simulink subsystem "Do_Model"  (R2022b)
settings: Solver=VariableStepAuto  StartTime=0.0  StopTime=10.0  RelTol=1e-3
undefined symbols (not defined in the file or in its folder): importedData
libraries: matrix_library x9
settings Model: Creator=hollis  LastModifiedBy=hollis

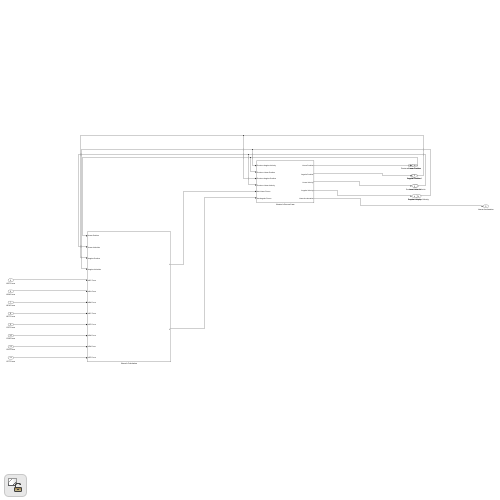
[thumbnail: Simulink's stored preview of the top-level diagram]
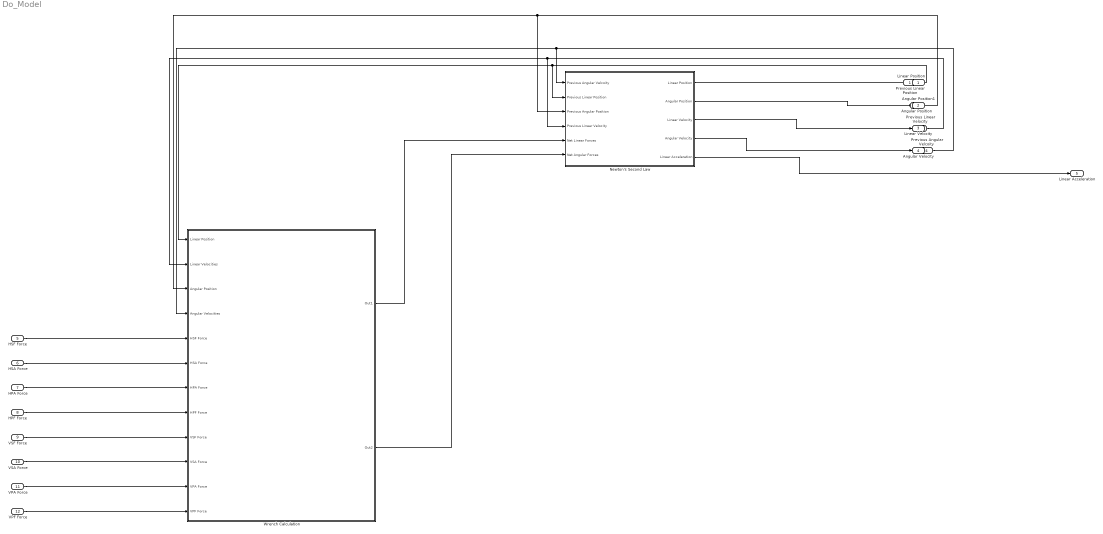
== system Do_Model ==
  Previous Linear Position : Inport
  Angular Position : Inport  Port=2
  Previous Linear Velocity : Inport  Port=3
  Previous Angular Velcoity : Inport  Port=4
  HSF Force : Inport  Port=5
  HSA Force : Inport  Port=6
  HPA Force : Inport  Port=7
  HPF Force : Inport  Port=8
  VSF Force : Inport  Port=9
  VSA Force : Inport  Port=10
  VPA Force : Inport  Port=11
  VPF Force : Inport  Port=12
  Newton's Second Law : Subsystem
  Wrench Calculation : Subsystem
  Linear Position : Outport
  Angular Position1 : Outport  Port=2
  Linear Velocity : Outport  Port=3
  Angular Velocity : Outport  Port=4
  Linear Acceleration : Outport  Port=5
  wires:
  VSF Force/1 -> Wrench Calculation/9(VSF Force)
  Newton's Second Law/3(Linear Velocity) -> Linear Velocity/1
  Wrench Calculation/2(Out2) -> Newton's Second Law/6(Net Angular Forces)
  Newton's Second Law/4(Angular Velocity) -> Angular Velocity/1
  VSA Force/1 -> Wrench Calculation/10(VSA Force)
  Wrench Calculation/1(Out1) -> Newton's Second Law/5(Net Linear Forces)
  HPA Force/1 -> Wrench Calculation/7(HPA Force)
  Previous Angular Velcoity/1 -> Wrench Calculation/4(Angular Velocities), Newton's Second Law/1(Previous Angular Velcoity)
  Newton's Second Law/2(Angular Position) -> Angular Position1/1
  HSA Force/1 -> Wrench Calculation/6(HSA Force)
  VPF Force/1 -> Wrench Calculation/12(VPF Force)
  VPA Force/1 -> Wrench Calculation/11(VPA Force)
  HSF Force/1 -> Wrench Calculation/5(HSF Force)
  Previous Linear Position/1 -> Wrench Calculation/1(Linear Position), Newton's Second Law/2(Previous Linear Position)
  Newton's Second Law/5(Linear Acceleration) -> Linear Acceleration/1
  Angular Position/1 -> Newton's Second Law/3(Previous Angular Position), Wrench Calculation/3(Angular Position)
  Newton's Second Law/1(Linear Position) -> Linear Position/1
  HPF Force/1 -> Wrench Calculation/8(HPF Force)
  Previous Linear Velocity/1 -> Wrench Calculation/2(Linear Velocities), Newton's Second Law/4(Previous Linear Velocity)

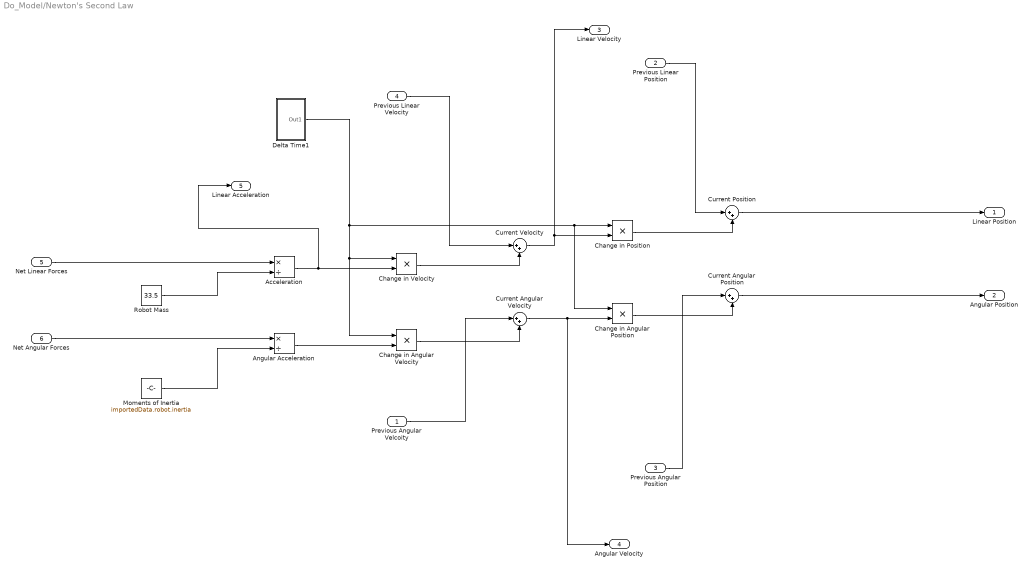
== system Do_Model/Newton's Second Law ==
  Previous Angular Velcoity : Inport
  Previous Linear Position : Inport  Port=2
  Previous Angular Position : Inport  Port=3
  Previous Linear Velocity : Inport  Port=4
  Net Linear Forces : Inport  Port=5
  Net Angular Forces : Inport  Port=6
  Acceleration : Product  Inputs=*/
  Angular Acceleration : Product  Inputs=*/
  Change in Angular Position : Product
  Change in Angular Velocity : Product
  Change in Position : Product
  Change in Velocity : Product
  Current Angular Position : Sum  Inputs=|++
  Current Angular Velocity : Sum  Inputs=|++
  Current Position : Sum  Inputs=|++
  Current Velocity : Sum  Inputs=|++
  Delta Time1 : Subsystem
  Moments of Inertia : Constant  Value=importedData.robot.inertia  VectorParams1D=off
  Robot Mass : Constant  Value=33.5
  Linear Position : Outport
  Angular Position : Outport  Port=2
  Linear Velocity : Outport  Port=3
  Angular Velocity : Outport  Port=4
  Linear Acceleration : Outport  Port=5
  wires:
  Change in Velocity/1 -> Current Velocity/2
  Previous Angular Position/1 -> Current Angular Position/1
  Robot Mass/1 -> Acceleration/2
  Previous Linear Position/1 -> Current Position/1
  Delta Time1/1(Out1) -> Change in Position/1, Change in Angular Position/1, Change in Velocity/1, Change in Angular Velocity/1
  Previous Angular Velcoity/1 -> Current Angular Velocity/1
  Change in Angular Position/1 -> Current Angular Position/2
  Current Angular Velocity/1 -> Change in Angular Position/2, Angular Velocity/1
  Net Angular Forces/1 -> Angular Acceleration/1
  Net Linear Forces/1 -> Acceleration/1
  Change in Angular Velocity/1 -> Current Angular Velocity/2
  Previous Linear Velocity/1 -> Current Velocity/1
  Current Position/1 -> Linear Position/1
  Current Velocity/1 -> Change in Position/2, Linear Velocity/1
  Moments of Inertia/1 -> Angular Acceleration/2
  Change in Position/1 -> Current Position/2
  Angular Acceleration/1 -> Change in Angular Velocity/2
  Acceleration/1 -> Change in Velocity/2, Linear Acceleration/1
  Current Angular Position/1 -> Angular Position/1

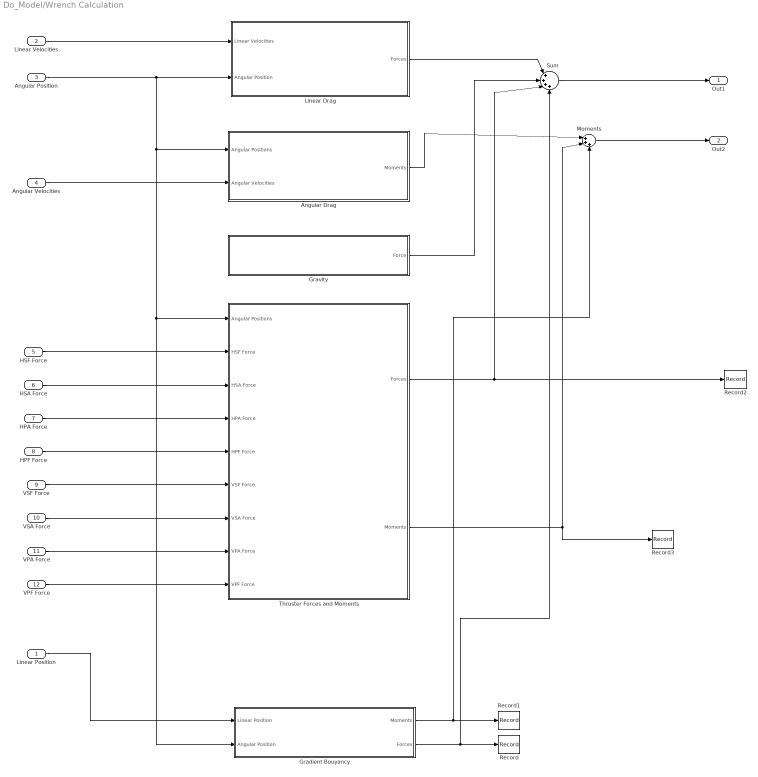
== system Do_Model/Wrench Calculation ==
  Linear Position : Inport
  Linear Velocities : Inport  Port=2
  Angular Position : Inport  Port=3
  Angular Velocities : Inport  Port=4
  HSF Force : Inport  Port=5
  HSA Force : Inport  Port=6
  HPA Force : Inport  Port=7
  HPF Force : Inport  Port=8
  VSF Force : Inport  Port=9
  VSA Force : Inport  Port=10
  VPA Force : Inport  Port=11
  VPF Force : Inport  Port=12
  Angular Drag : Subsystem
  Gradient Bouyancy : Subsystem
  Gravity : Subsystem
  Linear Drag : Subsystem
  Moments : Sum  Inputs=|+++
  Record : Record  FileSettingsInternal="{\"entries\":[{\"content\":{\"excelSettings\":{\"content\":{},\"type\":\"Streamout.ExcelSettings\"}},\"type\":\"Streamout.FileSettingStorage\",\"uuid\":\"413f287a-9b04-4e26-a977-dd89b3487b45\"}],\"packageUris\":[\"http://schema.mathworks.com/mf0/streamout_blocks/R2020a\"],\"version\":\"1.0\"}"  SignalsInternal="{\"entries\":[{\"content\":{\"signals\":[{\"content\":{\"blockPath\":[\"Do_Model/Wrench Calculation/Record\"],\"channel\":[],\"dimensions\":[1,3],\"domain\":\"Do_Model/Wrench Calculation/Record\",\"hasChildren\":true,\"lineColor\":\"#d95319\",\"plots\":[],\"port\":1,\"sid\":[],\"signalID\":1129,\"signalName\":\"Gradient Bouyancy:2\"},\"type\":\"RecordBlkView.Signal\",\"uuid\":\"34d04b5e-f248-43d4-9a10-f73c1ff918f2\"},{\"content\":{\"blockPath\":[\"Do_Model/Wrench Calculation/Record\"],\"channel\":[1,1],\"dimensions\":[1,3],\"domain\":\"Do_Model/Wrench Calculation/Record\",\"lineColor\":\"#ff6929\",\"parentID\":1129,\"plots\":[1],\"port\":1,\"sid\":[],\"signalID\":1130,\"signalName\":\"Gradient Bouyancy:2\"},\"type\":\"RecordBlkView.Signal\",\"uuid\":\"aa1ed0ec-f206-4fbe-a6ba-9fa76444e177\"},{\"content\":{\"blockPath\":[\"Do_Model/Wrench Calculation/Record\"],\"channel\":[1,2],\"dimensions\":[1,3],\"domain\":\"Do_Model/Wrench Calculation/Record\",\"lineColor\":\"#4dbeee\",\"parentID\":1129,\"plots\":[1],\"port\":1,\"sid\":[],\"signalID\":1131,\"signalName\":\"Gradient Bouyancy:2\"},\"type\":\"RecordBlkView.Signal\",\"uuid\":\"5ce51e6c-b958-4c9c-b847-18217f4c3a05\"},{\"content\":{\"blockPath\":[\"Do_Model/Wrench Calculation/Record\"],\"channel\":[1,3],\"dimensions\":[1,3],\"domain\":\"Do_Model/Wrench Calculation/Record\",\"lineColor\":\"#a2142f\",\"parentID\":1129,\"plots\":[1],\"port\":1,\"sid\":[],\"signalID\":1132,\"signalName\":\"Gradient Bouyancy:2\"},\"type\":\"RecordBlkView.Signal\",\"uuid\":\"1a67abd2-379e-4430-809d-af06210e5657\"}]},\"type\":\"RecordBlkView.InputSignals\",\"uuid\":\"051f222f-63c2-4983-ab2d-90b62d2a8a2a\"}],\"packageUris\":[\"http://schema.mathworks.com/mf0/streamout_blocks/R2020a\"],\"version\":\"1.0\"}"  VisualizationBindings="{\"sparklinesplugin\":{\"info\":[{\"bindingParametersList\":[],\"subplotID\":1}]}}"
  Record1 : Record  FileSettingsInternal="{\"entries\":[{\"content\":{\"excelSettings\":{\"content\":{},\"type\":\"Streamout.ExcelSettings\"}},\"type\":\"Streamout.FileSettingStorage\",\"uuid\":\"f64b510a-4950-46d7-a389-803d08724e03\"}],\"packageUris\":[\"http://schema.mathworks.com/mf0/streamout_blocks/R2020a\"],\"version\":\"1.0\"}"  SignalsInternal="{\"entries\":[{\"content\":{\"signals\":[{\"content\":{\"blockPath\":[\"Do_Model/Wrench Calculation/Record1\"],\"channel\":[],\"dimensions\":[1,3],\"domain\":\"Do_Model/Wrench Calculation/Record1\",\"hasChildren\":true,\"lineColor\":\"#7e2f8e\",\"plots\":[],\"port\":1,\"sid\":[],\"signalID\":1140,\"signalName\":\"Gradient Bouyancy:1\"},\"type\":\"RecordBlkView.Signal\",\"uuid\":\"a1cdf590-a143-44f5-92e8-d73606c7df01\"},{\"content\":{\"blockPath\":[\"Do_Model/Wrench Calculation/Record1\"],\"channel\":[1,1],\"dimensions\":[1,3],\"domain\":\"Do_Model/Wrench Calculation/Record1\",\"lineColor\":\"#64d413\",\"parentID\":1140,\"plots\":[1],\"port\":1,\"sid\":[],\"signalID\":1141,\"signalName\":\"Gradient Bouyancy:1\"},\"type\":\"RecordBlkView.Signal\",\"uuid\":\"417bb1a8-9de3-43e8-af8f-0c0af5ed7128\"},{\"content\":{\"blockPath\":[\"Do_Model/Wrench Calculation/Record1\"],\"channel\":[1,2],\"dimensions\":[1,3],\"domain\":\"Do_Model/Wrench Calculation/Record1\",\"lineColor\":\"#139fff\",\"parentID\":1140,\"plots\":[1],\"port\":1,\"sid\":[],\"signalID\":1142,\"signalName\":\"Gradient Bouyancy:1\"},\"type\":\"RecordBlkView.Signal\",\"uuid\":\"5a990a2d-a6b0-4250-bbb2-3801da7d4337\"},{\"content\":{\"blockPath\":[\"Do_Model/Wrench Calculation/Record1\"],\"channel\":[1,3],\"dimensions\":[1,3],\"domain\":\"Do_Model/Wrench Calculation/Record1\",\"lineColor\":\"#ff6929\",\"parentID\":1140,\"plots\":[1],\"port\":1,\"sid\":[],\"signalID\":1143,\"signalName\":\"Gradient Bouyancy:1\"},\"type\":\"RecordBlkView.Signal\",\"uuid\":\"b8287dae-b0e7-4c67-8bb2-6e8b0649e32a\"}]},\"type\":\"RecordBlkView.InputSignals\",\"uuid\":\"8bc7122d-09bb-47b7-8f1d-4618bb6a698e\"}],\"packageUris\":[\"http://schema.mathworks.com/mf0/streamout_blocks/R2020a\"],\"version\":\"1.0\"}"  VisualizationBindings="{\"sparklinesplugin\":{\"info\":[{\"bindingParametersList\":[],\"subplotID\":1}]}}"
  Record2 : Record  FileSettingsInternal="{\"entries\":[{\"content\":{\"excelSettings\":{\"content\":{},\"type\":\"Streamout.ExcelSettings\"}},\"type\":\"Streamout.FileSettingStorage\",\"uuid\":\"267244f1-9977-4a4c-80ac-3c245b9cb20c\"}],\"packageUris\":[\"http://schema.mathworks.com/mf0/streamout_blocks/R2020a\"],\"version\":\"1.0\"}"  SignalsInternal="{\"entries\":[{\"content\":{\"signals\":[{\"content\":{\"blockPath\":[\"Do_Model/Wrench Calculation/Record2\"],\"channel\":[],\"dimensions\":[1,3],\"domain\":\"Do_Model/Wrench Calculation/Record2\",\"hasChildren\":true,\"lineColor\":\"#4dbeee\",\"plots\":[],\"port\":1,\"sid\":[],\"signalID\":1151,\"signalName\":\"Thruster Forces and Moments:1\"},\"type\":\"RecordBlkView.Signal\",\"uuid\":\"8b4bdaab-6ae2-46b6-a3f9-3386a615984f\"},{\"content\":{\"blockPath\":[\"Do_Model/Wrench Calculation/Record2\"],\"channel\":[1,1],\"dimensions\":[1,3],\"domain\":\"Do_Model/Wrench Calculation/Record2\",\"lineColor\":\"#0072bd\",\"parentID\":1151,\"plots\":[1],\"port\":1,\"sid\":[],\"signalID\":1152,\"signalName\":\"Thruster Forces and Moments:1\"},\"type\":\"RecordBlkView.Signal\",\"uuid\":\"044b7272-3d90-4b5c-ac2a-024767f9643c\"},{\"content\":{\"blockPath\":[\"Do_Model/Wrench Calculation/Record2\"],\"channel\":[1,2],\"dimensions\":[1,3],\"domain\":\"Do_Model/Wrench Calculation/Record2\",\"lineColor\":\"#ff6929\",\"parentID\":1151,\"plots\":[1],\"port\":1,\"sid\":[],\"signalID\":1153,\"signalName\":\"Thruster Forces and Moments:1\"},\"type\":\"RecordBlkView.Signal\",\"uuid\":\"471c460b-d56a-4f0e-8ba6-626462a562e8\"},{\"content\":{\"blockPath\":[\"Do_Model/Wrench Calculation/Record2\"],\"channel\":[1,3],\"dimensions\":[1,3],\"domain\":\"Do_Model/Wrench Calculation/Record2\",\"lineColor\":\"#b746ff\",\"parentID\":1151,\"plots\":[1],\"port\":1,\"sid\":[],\"signalID\":1154,\"signalName\":\"Thruster Forces and Moments:1\"},\"type\":\"RecordBlkView.Signal\",\"uuid\":\"37346d9b-87df-428a-9c70-4b4edb3e39e8\"}]},\"type\":\"RecordBlkView.InputSignals\",\"uuid\":\"c9780bab-f0c1-411b-a2ab-d0ac7d34821e\"}],\"packageUris\":[\"http://schema.mathworks.com/mf0/streamout_blocks/R2020a\"],\"version\":\"1.0\"}"  VisualizationBindings="{\"sparklinesplugin\":{\"info\":[{\"bindingParametersList\":[],\"subplotID\":1}]}}"
  Record3 : Record  FileSettingsInternal="{\"entries\":[{\"content\":{\"excelSettings\":{\"content\":{},\"type\":\"Streamout.ExcelSettings\"}},\"type\":\"Streamout.FileSettingStorage\",\"uuid\":\"ea0166fd-875a-43db-b23d-202e0f7dcc7b\"}],\"packageUris\":[\"http://schema.mathworks.com/mf0/streamout_blocks/R2020a\"],\"version\":\"1.0\"}"  SignalsInternal="{\"entries\":[{\"content\":{\"signals\":[{\"content\":{\"blockPath\":[\"Do_Model/Wrench Calculation/Record3\"],\"channel\":[],\"dimensions\":[1,3],\"domain\":\"Do_Model/Wrench Calculation/Record3\",\"hasChildren\":true,\"lineColor\":\"#139fff\",\"plots\":[],\"port\":1,\"sid\":[],\"signalID\":1162,\"signalName\":\"Thruster Forces and Moments:2\"},\"type\":\"RecordBlkView.Signal\",\"uuid\":\"4842deb4-23c3-4b8f-af82-0d02d852bd5f\"},{\"content\":{\"blockPath\":[\"Do_Model/Wrench Calculation/Record3\"],\"channel\":[1,1],\"dimensions\":[1,3],\"domain\":\"Do_Model/Wrench Calculation/Record3\",\"lineColor\":\"#fe330a\",\"parentID\":1162,\"plots\":[1],\"port\":1,\"sid\":[],\"signalID\":1163,\"signalName\":\"Thruster Forces and Moments:2\"},\"type\":\"RecordBlkView.Signal\",\"uuid\":\"d1ebeda0-cc0e-41b9-9abc-3ddb45178fd5\"},{\"content\":{\"blockPath\":[\"Do_Model/Wrench Calculation/Record3\"],\"channel\":[1,2],\"dimensions\":[1,3],\"domain\":\"Do_Model/Wrench Calculation/Record3\",\"lineColor\":\"#fe330a\",\"parentID\":1162,\"plots\":[1],\"port\":1,\"sid\":[],\"signalID\":1164,\"signalName\":\"Thruster Forces and Moments:2\"},\"type\":\"RecordBlkView.Signal\",\"uuid\":\"f90ef1b5-80ea-494c-b7b4-60f9b5c38bf6\"},{\"content\":{\"blockPath\":[\"Do_Model/Wrench Calculation/Record3\"],\"channel\":[1,3],\"dimensions\":[1,3],\"domain\":\"Do_Model/Wrench Calculation/Record3\",\"lineColor\":\"#22b573\",\"parentID\":1162,\"plots\":[1],\"port\":1,\"sid\":[],\"signalID\":1165,\"signalName\":\"Thruster Forces and Moments:2\"},\"type\":\"RecordBlkView.Signal\",\"uuid\":\"b6e6d67f-9ddb-4794-ac0a-7bf0cc8401aa\"}]},\"type\":\"RecordBlkView.InputSignals\",\"uuid\":\"b8a63444-5f46-44cc-9b22-44435bccd4bb\"}],\"packageUris\":[\"http://schema.mathworks.com/mf0/streamout_blocks/R2020a\"],\"version\":\"1.0\"}"  VisualizationBindings="{\"sparklinesplugin\":{\"info\":[{\"bindingParametersList\":[],\"subplotID\":1}]}}"
  Sum : Sum  Inputs=|++++
  Thruster Forces and Moments : Subsystem
  Out1 : Outport
  Out2 : Outport  Port=2
  wires:
  Angular Velocities/1 -> Angular Drag/2(Angular Velocities)
  HPA Force/1 -> Thruster Forces and Moments/4(HPA Force)
  Linear Velocities/1 -> Linear Drag/1(Linear Velocities)
  VSF Force/1 -> Thruster Forces and Moments/6(VSF Force)
  Moments/1 -> Out2/1
  VPA Force/1 -> Thruster Forces and Moments/8(VPA Force)
  Gravity/1(Force) -> Sum/2
  HSA Force/1 -> Thruster Forces and Moments/3(HSA Force)
  HSF Force/1 -> Thruster Forces and Moments/2(HSF Force)
  VPF Force/1 -> Thruster Forces and Moments/9(VPF Force)
  HPF Force/1 -> Thruster Forces and Moments/5(HPF Force)
  Linear Drag/1(Forces) -> Sum/1
  Linear Position/1 -> Gradient Bouyancy/1(Linear Position)
  Angular Position/1 -> Thruster Forces and Moments/1(Angular Positions), Gradient Bouyancy/2(Angular Position), Angular Drag/1(Angular Positions), Linear Drag/2(Angular Position)
  Sum/1 -> Out1/1
  VSA Force/1 -> Thruster Forces and Moments/7(VSA Force)
  Gradient Bouyancy/1(Moments) -> Record1/1, Moments/3
  Gradient Bouyancy/2(Forces) -> Record/1, Sum/4
  Thruster Forces and Moments/2(Moments) -> Record3/1, Moments/2
  Angular Drag/1(Moments) -> Moments/1
  Thruster Forces and Moments/1(Forces) -> Sum/3, Record2/1

== system Do_Model/Newton's Second Law/Delta Time1 ==
  Clock : Clock
  Delta Time : Sum  Inputs=|+-
  Memory1 : Memory
  Out1 : Outport
  wires:
  Delta Time/1 -> Out1/1
  Clock/1 -> Delta Time/1, Memory1/1
  Memory1/1 -> Delta Time/2

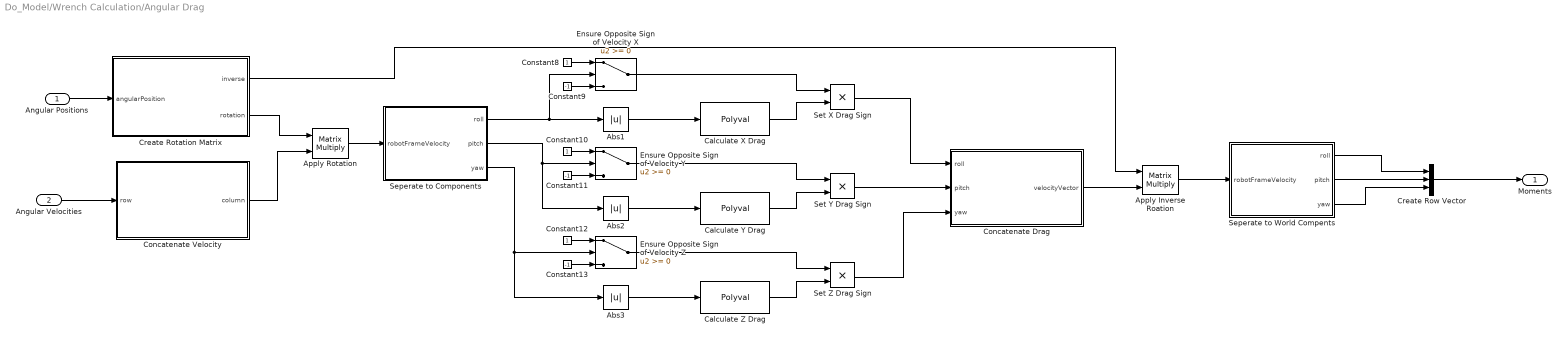
== system Do_Model/Wrench Calculation/Angular Drag ==
  Angular Positions : Inport
  Angular Velocities : Inport  Port=2
  Abs1 : Abs  SaturateOnIntegerOverflow=off
  Abs2 : Abs  SaturateOnIntegerOverflow=off
  Abs3 : Abs  SaturateOnIntegerOverflow=off
  Apply Inverse Roation : Product  Multiplication=Matrix(*)
  Apply Rotation : Product  Multiplication=Matrix(*)
  Calculate X Drag : Polyval  Coefs=importedData.robot.coefficients.roll
  Calculate Y Drag : Polyval  Coefs=importedData.robot.coefficients.pitch
  Calculate Z Drag : Polyval  Coefs=importedData.robot.coefficients.yaw
  Concatenate Drag : MATLAB Function  TreatAsAtomicUnit=on
  Concatenate Velocity : MATLAB Function  TreatAsAtomicUnit=on
  Constant10 : Constant
  Constant11 : Constant  Value=-1
  Constant12 : Constant
  Constant13 : Constant  Value=-1
  Constant8 : Constant
  Constant9 : Constant  Value=-1
  Create Rotation Matrix : MATLAB Function  TreatAsAtomicUnit=on
  Create Row Vector : Mux  Inputs=3
  Ensure Opposite Sign of Velocity X : Switch  SaturateOnIntegerOverflow=off  InputSameDT=off
  Ensure Opposite Sign of Velocity Y : Switch  SaturateOnIntegerOverflow=off  InputSameDT=off
  Ensure Opposite Sign of Velocity Z : Switch  SaturateOnIntegerOverflow=off  InputSameDT=off
  Seperate to Components : MATLAB Function  TreatAsAtomicUnit=on
  Seperate to World Compents : MATLAB Function  TreatAsAtomicUnit=on
  Set X Drag Sign : Product
  Set Y Drag Sign : Product
  Set Z Drag Sign : Product
  Moments : Outport
  wires:
  Angular Positions/1 -> Create Rotation Matrix/1(angularPosition)
  Create Row Vector/1 -> Moments/1
  Ensure Opposite Sign of Velocity Z/1 -> Set Z Drag Sign/1
  Seperate to Components/3(yaw) -> Abs3/1, Ensure Opposite Sign of Velocity Z/2
  Abs3/1 -> Calculate Z Drag/1
  Abs2/1 -> Calculate Y Drag/1
  Calculate X Drag/1 -> Set X Drag Sign/2
  Constant10/1 -> Ensure Opposite Sign of Velocity Y/1
  Create Rotation Matrix/1(inverse) -> Apply Inverse Roation/1
  Seperate to World Compents/2(pitch) -> Create Row Vector/2
  Seperate to Components/1(roll) -> Abs1/1, Ensure Opposite Sign of Velocity X/2
  Ensure Opposite Sign of Velocity X/1 -> Set X Drag Sign/1
  Seperate to World Compents/1(roll) -> Create Row Vector/1
  Concatenate Velocity/1(column) -> Apply Rotation/2
  Create Rotation Matrix/2(rotation) -> Apply Rotation/1
  Constant12/1 -> Ensure Opposite Sign of Velocity Z/1
  Seperate to World Compents/3(yaw) -> Create Row Vector/3
  Set X Drag Sign/1 -> Concatenate Drag/1(roll)
  Seperate to Components/2(pitch) -> Ensure Opposite Sign of Velocity Y/2, Abs2/1
  Ensure Opposite Sign of Velocity Y/1 -> Set Y Drag Sign/1
  Set Y Drag Sign/1 -> Concatenate Drag/2(pitch)
  Constant9/1 -> Ensure Opposite Sign of Velocity X/3
  Constant13/1 -> Ensure Opposite Sign of Velocity Z/3
  Set Z Drag Sign/1 -> Concatenate Drag/3(yaw)
  Constant8/1 -> Ensure Opposite Sign of Velocity X/1
  Angular Velocities/1 -> Concatenate Velocity/1(row)
  Apply Inverse Roation/1 -> Seperate to World Compents/1(robotFrameVelocity)
  Apply Rotation/1 -> Seperate to Components/1(robotFrameVelocity)
  Abs1/1 -> Calculate X Drag/1
  Calculate Z Drag/1 -> Set Z Drag Sign/2
  Constant11/1 -> Ensure Opposite Sign of Velocity Y/3
  Calculate Y Drag/1 -> Set Y Drag Sign/2
  Concatenate Drag/1(velocityVector) -> Apply Inverse Roation/2

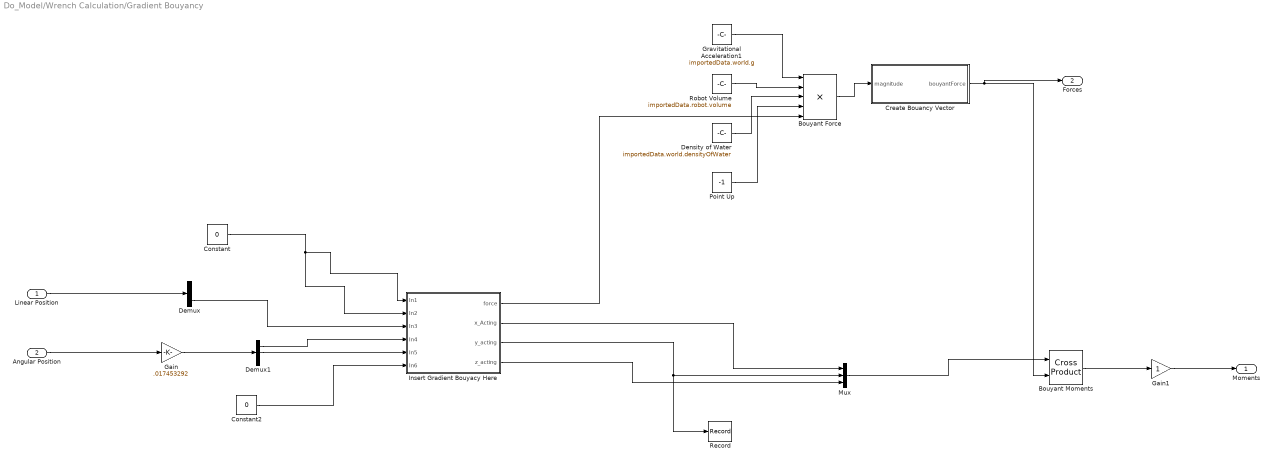
== system Do_Model/Wrench Calculation/Gradient Bouyancy ==
  Linear Position : Inport
  Angular Position : Inport  Port=2
  Bouyant Force : Product  Inputs=5
  Bouyant Moments : matrix_library/Cross Product
  Constant : Constant  Value=0
  Constant2 : Constant  Value=0
  Create Bouancy Vector : MATLAB Function  TreatAsAtomicUnit=on
  Demux : Demux  Outputs=3
  Demux1 : Demux  Outputs=3
  Density of Water : Constant  Value=importedData.world.densityOfWater
  Gain : Gain  Gain=.017453292
  Gain1 : Gain
  Gravitational Acceleration1 : Constant  Value=importedData.world.g
  Insert Gradient Bouyacy Here : Subsystem
  Mux : Mux  Inputs=3
  Point Up : Constant  Value=-1
  Record : Record  FileSettingsInternal="{\"entries\":[{\"content\":{\"excelSettings\":{\"content\":{},\"type\":\"Streamout.ExcelSettings\"}},\"type\":\"Streamout.FileSettingStorage\",\"uuid\":\"cfb1144b-3d43-4fc0-83f6-21f47d36b546\"}],\"packageUris\":[\"http://schema.mathworks.com/mf0/streamout_blocks/R2020a\"],\"version\":\"1.0\"}"  SignalsInternal="{\"entries\":[{\"content\":{\"signals\":[{\"content\":{\"blockPath\":[\"Do_Model/Wrench Calculation/Gradient Bouyancy/Record\"],\"channel\":[],\"dimensions\":[1,1],\"domain\":\"Do_Model/Wrench Calculation/Gradient Bouyancy/Record\",\"lineColor\":\"#7e2f8e\",\"plots\":[1],\"port\":1,\"sid\":[],\"signalID\":1124,\"signalName\":\"MATLAB System:3\"},\"type\":\"RecordBlkView.Signal\",\"uuid\":\"8ada3478-5f50-4bea-b160-c7958d3b34cc\"}]},\"type\":\"RecordBlkView.InputSignals\",\"uuid\":\"e34a299c-69e8-4726-acb2-46adb19b50a3\"}],\"packageUris\":[\"http://schema.mathworks.com/mf0/streamout_blocks/R2020a\"],\"version\":\"1.0\"}"  VisualizationBindings="{\"sparklinesplugin\":{\"info\":[{\"bindingParametersList\":[],\"subplotID\":1}]}}"
  Robot Volume : Constant  Value=importedData.robot.volume
  Moments : Outport
  Forces : Outport  Port=2
  wires:
  Constant/1 -> Insert Gradient Bouyacy Here/2(In2), Insert Gradient Bouyacy Here/1(In1)
  Linear Position/1 -> Demux/1
  Insert Gradient Bouyacy Here/4(z_acting) -> Mux/3
  Constant2/1 -> Insert Gradient Bouyacy Here/6(In6)
  Gain1/1 -> Moments/1
  Gain/1 -> Demux1/1
  Insert Gradient Bouyacy Here/3(y_acting) -> Mux/2, Record/1
  Insert Gradient Bouyacy Here/2(x_Acting) -> Mux/1
  Mux/1 -> Bouyant Moments/1
  Demux1/2 -> Insert Gradient Bouyacy Here/5(In5)
  Demux1/1 -> Insert Gradient Bouyacy Here/4(In4)
  Angular Position/1 -> Gain/1
  Demux/3 -> Insert Gradient Bouyacy Here/3(In3)
  Insert Gradient Bouyacy Here/1(force) -> Bouyant Force/5
  Point Up/1 -> Bouyant Force/4
  Bouyant Moments/1 -> Gain1/1
  Robot Volume/1 -> Bouyant Force/2
  Create Bouancy Vector/1(bouyantForce) -> Forces/1, Bouyant Moments/2
  Bouyant Force/1 -> Create Bouancy Vector/1(magnitude)
  Gravitational Acceleration1/1 -> Bouyant Force/1
  Density of Water/1 -> Bouyant Force/3

== system Do_Model/Wrench Calculation/Gravity ==
  Create Vector : MATLAB Function  TreatAsAtomicUnit=on
  Gravitational Acceleration1 : Constant  Value=importedData.world.g
  Gravitational Force1 : Product
  Robot Mass : Constant  Value=33.5
  Force : Outport
  wires:
  Gravitational Force1/1 -> Create Vector/1(magnitude)
  Create Vector/1(vector) -> Force/1
  Robot Mass/1 -> Gravitational Force1/2
  Gravitational Acceleration1/1 -> Gravitational Force1/1

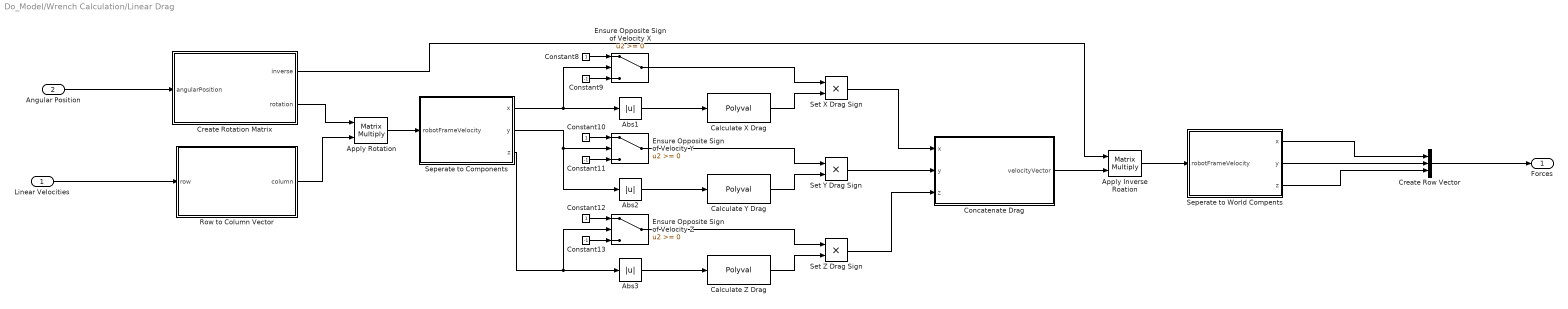
== system Do_Model/Wrench Calculation/Linear Drag ==
  Linear Velocities : Inport
  Angular Position : Inport  Port=2
  Abs1 : Abs  SaturateOnIntegerOverflow=off
  Abs2 : Abs  SaturateOnIntegerOverflow=off
  Abs3 : Abs  SaturateOnIntegerOverflow=off
  Apply Inverse Roation : Product  Multiplication=Matrix(*)
  Apply Rotation : Product  Multiplication=Matrix(*)
  Calculate X Drag : Polyval  Coefs=importedData.robot.coefficients.x
  Calculate Y Drag : Polyval  Coefs=importedData.robot.coefficients.y
  Calculate Z Drag : Polyval  Coefs=importedData.robot.coefficients.z
  Concatenate Drag : MATLAB Function  TreatAsAtomicUnit=on
  Constant10 : Constant
  Constant11 : Constant  Value=-1
  Constant12 : Constant
  Constant13 : Constant  Value=-1
  Constant8 : Constant
  Constant9 : Constant  Value=-1
  Create Rotation Matrix : MATLAB Function  TreatAsAtomicUnit=on
  Create Row Vector : Mux  Inputs=3
  Ensure Opposite Sign of Velocity X : Switch  SaturateOnIntegerOverflow=off  InputSameDT=off
  Ensure Opposite Sign of Velocity Y : Switch  SaturateOnIntegerOverflow=off  InputSameDT=off
  Ensure Opposite Sign of Velocity Z : Switch  SaturateOnIntegerOverflow=off  InputSameDT=off
  Row to Column Vector : MATLAB Function  TreatAsAtomicUnit=on
  Seperate to Components : MATLAB Function  TreatAsAtomicUnit=on
  Seperate to World Compents : MATLAB Function  TreatAsAtomicUnit=on
  Set X Drag Sign : Product
  Set Y Drag Sign : Product
  Set Z Drag Sign : Product
  Forces : Outport
  wires:
  Linear Velocities/1 -> Row to Column Vector/1(row)
  Create Row Vector/1 -> Forces/1
  Seperate to World Compents/3(z) -> Create Row Vector/3
  Seperate to World Compents/1(x) -> Create Row Vector/1
  Seperate to World Compents/2(y) -> Create Row Vector/2
  Ensure Opposite Sign of Velocity Z/1 -> Set Z Drag Sign/1
  Set X Drag Sign/1 -> Concatenate Drag/1(x)
  Set Y Drag Sign/1 -> Concatenate Drag/2(y)
  Ensure Opposite Sign of Velocity Y/1 -> Set Y Drag Sign/1
  Angular Position/1 -> Create Rotation Matrix/1(angularPosition)
  Calculate Z Drag/1 -> Set Z Drag Sign/2
  Apply Rotation/1 -> Seperate to Components/1(robotFrameVelocity)
  Constant11/1 -> Ensure Opposite Sign of Velocity Y/3
  Seperate to Components/1(x) -> Ensure Opposite Sign of Velocity X/2, Abs1/1
  Seperate to Components/2(y) -> Ensure Opposite Sign of Velocity Y/2, Abs2/1
  Constant10/1 -> Ensure Opposite Sign of Velocity Y/1
  Row to Column Vector/1(column) -> Apply Rotation/2
  Create Rotation Matrix/2(rotation) -> Apply Rotation/1
  Create Rotation Matrix/1(inverse) -> Apply Inverse Roation/1
  Constant13/1 -> Ensure Opposite Sign of Velocity Z/3
  Constant9/1 -> Ensure Opposite Sign of Velocity X/3
  Apply Inverse Roation/1 -> Seperate to World Compents/1(robotFrameVelocity)
  Calculate Y Drag/1 -> Set Y Drag Sign/2
  Concatenate Drag/1(velocityVector) -> Apply Inverse Roation/2
  Abs1/1 -> Calculate X Drag/1
  Abs3/1 -> Calculate Z Drag/1
  Set Z Drag Sign/1 -> Concatenate Drag/3(z)
  Seperate to Components/3(z) -> Ensure Opposite Sign of Velocity Z/2, Abs3/1
  Constant8/1 -> Ensure Opposite Sign of Velocity X/1
  Abs2/1 -> Calculate Y Drag/1
  Constant12/1 -> Ensure Opposite Sign of Velocity Z/1
  Ensure Opposite Sign of Velocity X/1 -> Set X Drag Sign/1
  Calculate X Drag/1 -> Set X Drag Sign/2

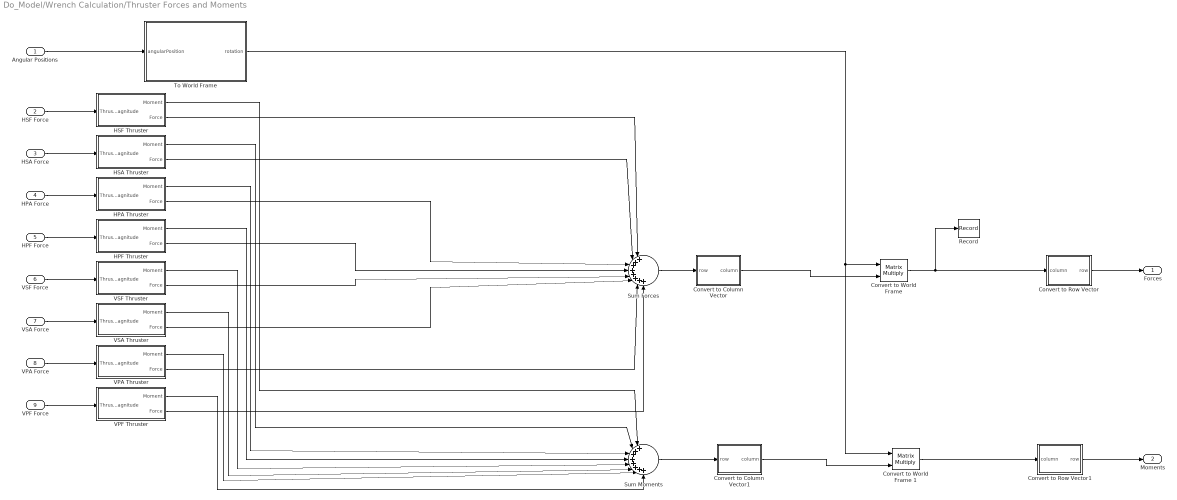
== system Do_Model/Wrench Calculation/Thruster Forces and Moments ==
  Angular Positions : Inport
  HSF Force : Inport  Port=2
  HSA Force : Inport  Port=3
  HPA Force : Inport  Port=4
  HPF Force : Inport  Port=5
  VSF Force : Inport  Port=6
  VSA Force : Inport  Port=7
  VPA Force : Inport  Port=8
  VPF Force : Inport  Port=9
  Convert to Column Vector : MATLAB Function  TreatAsAtomicUnit=on
  Convert to Column Vector1 : MATLAB Function  TreatAsAtomicUnit=on
  Convert to Row Vector : MATLAB Function  TreatAsAtomicUnit=on
  Convert to Row Vector1 : MATLAB Function  TreatAsAtomicUnit=on
  Convert to World Frame : Product  Multiplication=Matrix(*)
  Convert to World Frame 1 : Product  Multiplication=Matrix(*)
  HPA Thruster : Subsystem
  HPF Thruster : Subsystem
  HSA Thruster : Subsystem
  HSF Thruster : Subsystem
  Record : Record  FileSettingsInternal="{\"entries\":[{\"content\":{\"excelSettings\":{\"content\":{},\"type\":\"Streamout.ExcelSettings\"}},\"type\":\"Streamout.FileSettingStorage\",\"uuid\":\"0b1fec21-7c3d-44ca-be35-70baeb02196c\"}],\"packageUris\":[\"http://schema.mathworks.com/mf0/streamout_blocks/R2020a\"],\"version\":\"1.0\"}"  SignalsInternal="{\"entries\":[{\"content\":{\"signals\":[{\"content\":{\"blockPath\":[\"Do_Model/Wrench Calculation/Thruster Forces and Moments/Record\"],\"channel\":[],\"dimensions\":[3,1],\"domain\":\"Do_Model/Wrench Calculation/Thruster Forces and Moments/Record\",\"hasChildren\":true,\"lineColor\":\"#64d413\",\"plots\":[],\"port\":1,\"sid\":[],\"signalID\":1173,\"signalName\":\"Convert to World Frame\"},\"type\":\"RecordBlkView.Signal\",\"uuid\":\"34468a32-5a30-45d9-9b27-f6383c81ce87\"},{\"content\":{\"blockPath\":[\"Do_Model/Wrench Calculation/Thruster Forces and Moments/Record\"],\"channel\":[1,1],\"dimensions\":[3,1],\"domain\":\"Do_Model/Wrench Calculation/Thruster Forces and Moments/Record\",\"lineColor\":\"#a2142f\",\"parentID\":1173,\"plots\":[1],\"port\":1,\"sid\":[],\"signalID\":1174,\"signalName\":\"Convert to World Frame\"},\"type\":\"RecordBlkView.Signal\",\"uuid\":\"7e516d3e-4349-4ac6-a75e-d81d97c1859e\"},{\"content\":{\"blockPath\":[\"Do_Model/Wrench Calculation/Thruster Forces and Moments/Record\"],\"channel\":[2,1],\"dimensions\":[3,1],\"domain\":\"Do_Model/Wrench Calculation/Thruster Forces and Moments/Record\",\"lineColor\":\"#ff13a6\",\"parentID\":1173,\"plots\":[1],\"port\":1,\"sid\":[],\"signalID\":1175,\"signalName\":\"Convert to World Frame\"},\"type\":\"RecordBlkView.Signal\",\"uuid\":\"efd14404-b3c3-4b7e-a343-39f1f57b2a06\"},{\"content\":{\"blockPath\":[\"Do_Model/Wrench Calculation/Thruster Forces and Moments/Record\"],\"channel\":[3,1],\"dimensions\":[3,1],\"domain\":\"Do_Model/Wrench Calculation/Thruster Forces and Moments/Record\",\"lineColor\":\"#fe330a\",\"parentID\":1173,\"plots\":[1],\"port\":1,\"sid\":[],\"signalID\":1176,\"signalName\":\"Convert to World Frame\"},\"type\":\"RecordBlkView.Signal\",\"uuid\":\"ceba797a-39b8-45ed-b5e6-e690261baff2\"}]},\"type\":\"RecordBlkView.InputSignals\",\"uuid\":\"ae40bfe1-a69a-4f79-ac02-c222108892d7\"}],\"packageUris\":[\"http://schema.mathworks.com/mf0/streamout_blocks/R2020a\"],\"version\":\"1.0\"}"  VisualizationBindings="{\"sparklinesplugin\":{\"info\":[{\"bindingParametersList\":[],\"subplotID\":1}]}}"
  Sum Forces : Sum  Inputs=|++++++++  InputSameDT=on
  Sum Moments : Sum  Inputs=|++++++++
  To World Frame : MATLAB Function  TreatAsAtomicUnit=on
  VPA Thruster : Subsystem
  VPF Thruster : Subsystem
  VSA Thruster : Subsystem
  VSF Thruster : Subsystem
  Forces : Outport
  Moments : Outport  Port=2
  wires:
  Sum Moments/1 -> Convert to Column Vector1/1(row)
  Convert to Column Vector1/1(column) -> Convert to World Frame 1/2
  Convert to Row Vector1/1(row) -> Moments/1
  Convert to World Frame 1/1 -> Convert to Row Vector1/1(column)
  To World Frame/1(rotation) -> Convert to World Frame/1, Convert to World Frame 1/1
  Convert to World Frame/1 -> Convert to Row Vector/1(column), Record/1
  Convert to Column Vector/1(column) -> Convert to World Frame/2
  Convert to Row Vector/1(row) -> Forces/1
  Angular Positions/1 -> To World Frame/1(angularPosition)
  VSA Thruster/1(Moment) -> Sum Moments/6
  VPF Thruster/2(Force) -> Sum Forces/8
  HSA Force/1 -> HSA Thruster/1(Thrust Magnitude)
  VPA Thruster/1(Moment) -> Sum Moments/7
  HPA Force/1 -> HPA Thruster/1(Thrust Magnitude)
  HSF Thruster/2(Force) -> Sum Forces/1
  Sum Forces/1 -> Convert to Column Vector/1(row)
  HPA Thruster/2(Force) -> Sum Forces/3
  VPA Thruster/2(Force) -> Sum Forces/7
  HPF Force/1 -> HPF Thruster/1(Thrust Magnitude)
  VSA Force/1 -> VSA Thruster/1(Thrust Magnitude)
  HSA Thruster/2(Force) -> Sum Forces/2
  VPF Thruster/1(Moment) -> Sum Moments/8
  VPF Force/1 -> VPF Thruster/1(Thrust Magnitude)
  VPA Force/1 -> VPA Thruster/1(Thrust Magnitude)
  HPF Thruster/1(Moment) -> Sum Moments/4
  VSA Thruster/2(Force) -> Sum Forces/6
  HSA Thruster/1(Moment) -> Sum Moments/2
  HPF Thruster/2(Force) -> Sum Forces/4
  VSF Force/1 -> VSF Thruster/1(Thrust Magnitude)
  HPA Thruster/1(Moment) -> Sum Moments/3
  VSF Thruster/1(Moment) -> Sum Moments/5
  HSF Force/1 -> HSF Thruster/1(Thrust Magnitude)
  HSF Thruster/1(Moment) -> Sum Moments/1
  VSF Thruster/2(Force) -> Sum Forces/5

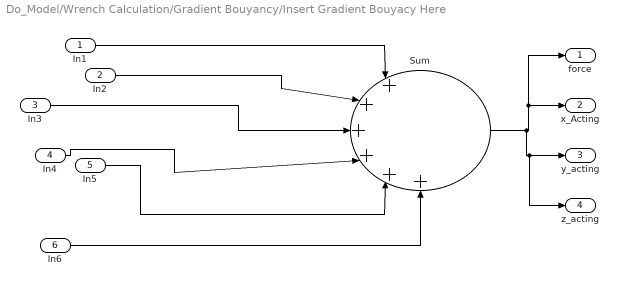
== system Do_Model/Wrench Calculation/Gradient Bouyancy/Insert Gradient Bouyacy Here ==
  In1 : Inport
  In2 : Inport  Port=2
  In3 : Inport  Port=3
  In4 : Inport  Port=4
  In5 : Inport  Port=5
  In6 : Inport  Port=6
  Sum : Sum  Inputs=|++++++
  force : Outport
  x_Acting : Outport  Port=2
  y_acting : Outport  Port=3
  z_acting : Outport  Port=4
  wires:
  Sum/1 -> force/1, x_Acting/1, y_acting/1, z_acting/1
  In1/1 -> Sum/1
  In6/1 -> Sum/6
  In4/1 -> Sum/4
  In3/1 -> Sum/3
  In2/1 -> Sum/2
  In5/1 -> Sum/5

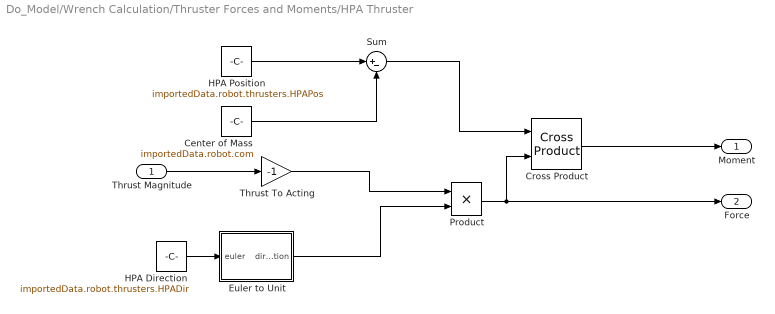
== system Do_Model/Wrench Calculation/Thruster Forces and Moments/HPA Thruster ==
  Thrust Magnitude : Inport
  Center of Mass : Constant  Value=importedData.robot.com
  Cross Product : matrix_library/Cross Product
  Euler to Unit : MATLAB Function  TreatAsAtomicUnit=on
  HPA Direction : Constant  Value=importedData.robot.thrusters.HPADir  VectorParams1D=off
  HPA Position : Constant  Value=importedData.robot.thrusters.HPAPos  VectorParams1D=off
  Product : Product
  Sum : Sum  Inputs=|+-
  Thrust To Acting : Gain  Gain=-1
  Moment : Outport
  Force : Outport  Port=2
  wires:
  Thrust To Acting/1 -> Product/1
  Sum/1 -> Cross Product/1
  Center of Mass/1 -> Sum/2
  HPA Position/1 -> Sum/1
  Euler to Unit/1(direction) -> Product/2
  HPA Direction/1 -> Euler to Unit/1(euler)
  Thrust Magnitude/1 -> Thrust To Acting/1
  Cross Product/1 -> Moment/1
  Product/1 -> Cross Product/2, Force/1

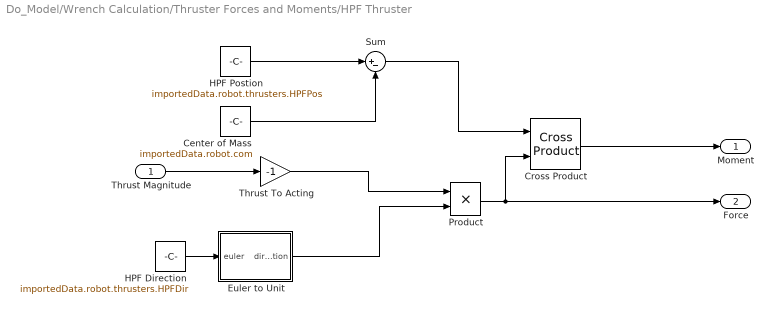
== system Do_Model/Wrench Calculation/Thruster Forces and Moments/HPF Thruster ==
  Thrust Magnitude : Inport
  Center of Mass : Constant  Value=importedData.robot.com
  Cross Product : matrix_library/Cross Product
  Euler to Unit : MATLAB Function  TreatAsAtomicUnit=on
  HPF Direction : Constant  Value=importedData.robot.thrusters.HPFDir  VectorParams1D=off
  HPF Postion : Constant  Value=importedData.robot.thrusters.HPFPos  VectorParams1D=off
  Product : Product
  Sum : Sum  Inputs=|+-
  Thrust To Acting : Gain  Gain=-1
  Moment : Outport
  Force : Outport  Port=2
  wires:
  Thrust To Acting/1 -> Product/1
  Sum/1 -> Cross Product/1
  Center of Mass/1 -> Sum/2
  HPF Postion/1 -> Sum/1
  Euler to Unit/1(direction) -> Product/2
  HPF Direction/1 -> Euler to Unit/1(euler)
  Thrust Magnitude/1 -> Thrust To Acting/1
  Cross Product/1 -> Moment/1
  Product/1 -> Cross Product/2, Force/1

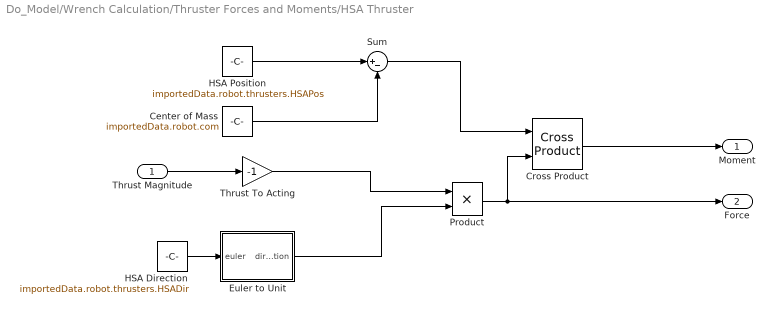
== system Do_Model/Wrench Calculation/Thruster Forces and Moments/HSA Thruster ==
  Thrust Magnitude : Inport
  Center of Mass : Constant  Value=importedData.robot.com
  Cross Product : matrix_library/Cross Product
  Euler to Unit : MATLAB Function  TreatAsAtomicUnit=on
  HSA Direction : Constant  Value=importedData.robot.thrusters.HSADir  VectorParams1D=off
  HSA Position : Constant  Value=importedData.robot.thrusters.HSAPos  VectorParams1D=off
  Product : Product
  Sum : Sum  Inputs=|+-
  Thrust To Acting : Gain  Gain=-1
  Moment : Outport
  Force : Outport  Port=2
  wires:
  Thrust To Acting/1 -> Product/1
  Sum/1 -> Cross Product/1
  Center of Mass/1 -> Sum/2
  HSA Position/1 -> Sum/1
  Euler to Unit/1(direction) -> Product/2
  HSA Direction/1 -> Euler to Unit/1(euler)
  Thrust Magnitude/1 -> Thrust To Acting/1
  Cross Product/1 -> Moment/1
  Product/1 -> Cross Product/2, Force/1

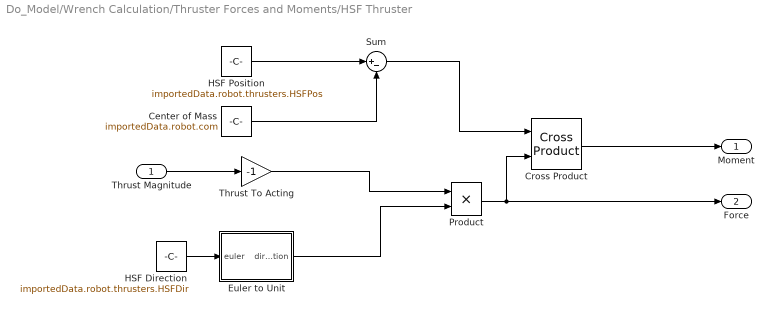
== system Do_Model/Wrench Calculation/Thruster Forces and Moments/HSF Thruster ==
  Thrust Magnitude : Inport
  Center of Mass : Constant  Value=importedData.robot.com
  Cross Product : matrix_library/Cross Product
  Euler to Unit : MATLAB Function  TreatAsAtomicUnit=on
  HSF Direction : Constant  Value=importedData.robot.thrusters.HSFDir  VectorParams1D=off
  HSF Position : Constant  Value=importedData.robot.thrusters.HSFPos  VectorParams1D=off
  Product : Product
  Sum : Sum  Inputs=|+-
  Thrust To Acting : Gain  Gain=-1
  Moment : Outport
  Force : Outport  Port=2
  wires:
  Thrust To Acting/1 -> Product/1
  Sum/1 -> Cross Product/1
  Center of Mass/1 -> Sum/2
  HSF Position/1 -> Sum/1
  Euler to Unit/1(direction) -> Product/2
  HSF Direction/1 -> Euler to Unit/1(euler)
  Thrust Magnitude/1 -> Thrust To Acting/1
  Cross Product/1 -> Moment/1
  Product/1 -> Cross Product/2, Force/1

== system Do_Model/Wrench Calculation/Thruster Forces and Moments/VPA Thruster ==
  Thrust Magnitude : Inport
  Center of Mass : Constant  Value=importedData.robot.com
  Cross Product : matrix_library/Cross Product
  Euler to Unit : MATLAB Function  TreatAsAtomicUnit=on
  Product : Product
  Sum : Sum  Inputs=|+-
  Thrust To Acting : Gain  Gain=-1
  VPA Direction : Constant  Value=importedData.robot.thrusters.VPADir  VectorParams1D=off
  VPA Position : Constant  Value=importedData.robot.thrusters.VPAPos  VectorParams1D=off
  Moment : Outport
  Force : Outport  Port=2
  wires:
  Thrust To Acting/1 -> Product/1
  Sum/1 -> Cross Product/1
  Center of Mass/1 -> Sum/2
  VPA Position/1 -> Sum/1
  Euler to Unit/1(direction) -> Product/2
  VPA Direction/1 -> Euler to Unit/1(euler)
  Thrust Magnitude/1 -> Thrust To Acting/1
  Cross Product/1 -> Moment/1
  Product/1 -> Cross Product/2, Force/1

== system Do_Model/Wrench Calculation/Thruster Forces and Moments/VPF Thruster ==
  Thrust Magnitude : Inport
  Center of Mass : Constant  Value=importedData.robot.com
  Cross Product : matrix_library/Cross Product
  Euler to Unit : MATLAB Function  TreatAsAtomicUnit=on
  Product : Product
  Sum : Sum  Inputs=|+-
  Thrust To Acting : Gain  Gain=-1
  VPF Direction : Constant  Value=importedData.robot.thrusters.VPFDir  VectorParams1D=off
  VPF Position : Constant  Value=importedData.robot.thrusters.VPFPos  VectorParams1D=off
  Moment : Outport
  Force : Outport  Port=2
  wires:
  Thrust To Acting/1 -> Product/1
  Sum/1 -> Cross Product/1
  Center of Mass/1 -> Sum/2
  VPF Position/1 -> Sum/1
  Euler to Unit/1(direction) -> Product/2
  VPF Direction/1 -> Euler to Unit/1(euler)
  Thrust Magnitude/1 -> Thrust To Acting/1
  Cross Product/1 -> Moment/1
  Product/1 -> Cross Product/2, Force/1

== system Do_Model/Wrench Calculation/Thruster Forces and Moments/VSA Thruster ==
  Thrust Magnitude : Inport
  Center of Mass : Constant  Value=importedData.robot.com
  Cross Product : matrix_library/Cross Product
  Euler to Unit : MATLAB Function  TreatAsAtomicUnit=on
  Product : Product
  Sum : Sum  Inputs=|+-
  Thrust To Acting : Gain  Gain=-1
  VSA Direction : Constant  Value=importedData.robot.thrusters.VSADir  VectorParams1D=off
  VSA Position : Constant  Value=importedData.robot.thrusters.VSAPos  VectorParams1D=off
  Moment : Outport
  Force : Outport  Port=2
  wires:
  Thrust To Acting/1 -> Product/1
  Sum/1 -> Cross Product/1
  Center of Mass/1 -> Sum/2
  VSA Position/1 -> Sum/1
  Euler to Unit/1(direction) -> Product/2
  VSA Direction/1 -> Euler to Unit/1(euler)
  Thrust Magnitude/1 -> Thrust To Acting/1
  Cross Product/1 -> Moment/1
  Product/1 -> Cross Product/2, Force/1

== system Do_Model/Wrench Calculation/Thruster Forces and Moments/VSF Thruster ==
  Thrust Magnitude : Inport
  Center of Mass : Constant  Value=importedData.robot.com
  Cross Product : matrix_library/Cross Product
  Euler to Unit : MATLAB Function  TreatAsAtomicUnit=on
  Product : Product
  Sum : Sum  Inputs=|+-
  Thrust To Acting : Gain  Gain=-1
  VSF Direction : Constant  Value=importedData.robot.thrusters.VSFDir  VectorParams1D=off
  VSF Position : Constant  Value=importedData.robot.thrusters.VSFPos  VectorParams1D=off
  Moment : Outport
  Force : Outport  Port=2
  wires:
  Thrust To Acting/1 -> Product/1
  Sum/1 -> Cross Product/1
  Center of Mass/1 -> Sum/2
  VSF Position/1 -> Sum/1
  Euler to Unit/1(direction) -> Product/2
  VSF Direction/1 -> Euler to Unit/1(euler)
  Thrust Magnitude/1 -> Thrust To Acting/1
  Cross Product/1 -> Moment/1
  Product/1 -> Cross Product/2, Force/1

== matlab function Do_Model/Wrench Calculation/Linear Drag/Row to Column Vector ==
  data: row input; column output
function column = fcn(row)

column = [row(1); row(2); row(3)];

== matlab function Do_Model/Wrench Calculation/Thruster Forces and Moments/HSA Thruster/Euler to Unit ==
  data: euler input; direction output
function direction = fcn(euler)

directionCol = eul2rotm(euler, "XYZ") * [1; 0; 0];
direction = [directionCol(1,1), directionCol(2,1), directionCol(3,1)];

== matlab function Do_Model/Wrench Calculation/Thruster Forces and Moments/HPA Thruster/Euler to Unit ==
  data: euler input; direction output
function direction = fcn(euler)

directionCol = eul2rotm(euler, "XYZ") * [1; 0; 0];
direction = [directionCol(1,1), directionCol(2,1), directionCol(3,1)];

== matlab function Do_Model/Wrench Calculation/Thruster Forces and Moments/HPF Thruster/Euler to Unit ==
  data: euler input; direction output
function direction = fcn(euler)

directionCol = eul2rotm(euler, "XYZ") * [1; 0; 0];
direction = [directionCol(1,1), directionCol(2,1), directionCol(3,1)];

== matlab function Do_Model/Wrench Calculation/Thruster Forces and Moments/VSF Thruster/Euler to Unit ==
  data: euler input; direction output
function direction = fcn(euler)

directionCol = eul2rotm(euler, "XYZ") * [1; 0; 0];
direction = [directionCol(1,1), directionCol(2,1), directionCol(3,1)];

== matlab function Do_Model/Wrench Calculation/Thruster Forces and Moments/VSA Thruster/Euler to Unit ==
  data: euler input; direction output
function direction = fcn(euler)

directionCol = eul2rotm(euler, "XYZ") * [1; 0; 0];
direction = [directionCol(1,1), directionCol(2,1), directionCol(3,1)];

== matlab function Do_Model/Wrench Calculation/Thruster Forces and Moments/VPA Thruster/Euler to Unit ==
  data: euler input; direction output
function direction = fcn(euler)

directionCol = eul2rotm(euler, "XYZ") * [1; 0; 0];
direction = [directionCol(1,1), directionCol(2,1), directionCol(3,1)];

== matlab function Do_Model/Wrench Calculation/Thruster Forces and Moments/VPF Thruster/Euler to Unit ==
  data: euler input; direction output
function direction = fcn(euler)

directionCol = eul2rotm(euler, "XYZ") * [1; 0; 0];
direction = [directionCol(1,1), directionCol(2,1), directionCol(3,1)];

== matlab function Do_Model/Wrench Calculation/Gravity/Create Vector ==
  data: magnitude input; vector output
function vector = fcn(magnitude)

vector = [0, 0, magnitude];

== matlab function Do_Model/Wrench Calculation/Thruster Forces and Moments/To World Frame ==
  data: angularPosition input; rotation output
function rotation  = fcn(angularPosition)

rotationToRobot = eul2rotm([deg2rad(angularPosition(1)), deg2rad(angularPosition(2)), deg2rad(angularPosition(3))]); %create the rotation matrix to robot frame

rotation = transpose(rotationToRobot);

== matlab function Do_Model/Wrench Calculation/Thruster Forces and Moments/Convert to Column Vector ==
  data: row input; column output
function column = fcn(row)

column = [row(1); row(2); row(3)];

== matlab function Do_Model/Wrench Calculation/Linear Drag/Create Rotation Matrix ==
  data: inverse output; angularPosition input; rotation output
function [inverse, rotation] = fcn(angularPosition)

rotation = eul2rotm([deg2rad(angularPosition(1)), deg2rad(angularPosition(2)), deg2rad(angularPosition(3))]);
inverse = transpose(rotation);

== matlab function Do_Model/Wrench Calculation/Thruster Forces and Moments/Convert to Row Vector ==
  data: column input; row output
function row = fcn(column)

row = [column(1,1), column(2,1), column(3,1)];

== matlab function Do_Model/Wrench Calculation/Thruster Forces and Moments/Convert to Column Vector1 ==
  data: row input; column output
function column = fcn(row)

column = [row(1); row(2); row(3)];

== matlab function Do_Model/Wrench Calculation/Thruster Forces and Moments/Convert to Row Vector1 ==
  data: column input; row output
function row = fcn(column)

row = [column(1,1), column(2,1), column(3,1)];

== matlab function Do_Model/Wrench Calculation/Gradient Bouyancy/Create Bouancy Vector ==
  data: magnitude input; bouyantForce output
function bouyantForce = fcn(magnitude)

bouyantForce = [0, 0, magnitude];

== matlab function Do_Model/Wrench Calculation/Linear Drag/Seperate to Components ==
  data: x output; robotFrameVelocity input; y output; z output
function [x, y, z] = fcn(robotFrameVelocity)

x = robotFrameVelocity(1, 1);
y = robotFrameVelocity(2, 1);
z = robotFrameVelocity(3, 1);

== matlab function Do_Model/Wrench Calculation/Linear Drag/Concatenate Drag ==
  data: x input; velocityVector output; y input; z input
function velocityVector = fcn(x,y,z)

velocityVector = [x; y; z];

== matlab function Do_Model/Wrench Calculation/Linear Drag/Seperate to World Compents ==
  data: x output; robotFrameVelocity input; y output; z output
function [x, y, z] = fcn(robotFrameVelocity)

x = robotFrameVelocity(1, 1);
y = robotFrameVelocity(2, 1);
z = robotFrameVelocity(3, 1);

== matlab function Do_Model/Wrench Calculation/Angular Drag/Concatenate Drag ==
  data: roll input; velocityVector output; pitch input; yaw input
function velocityVector = fcn(roll,pitch,yaw)

velocityVector = [roll; pitch; yaw];

== matlab function Do_Model/Wrench Calculation/Angular Drag/Concatenate Velocity ==
  data: row input; column output
function column = fcn(row)

column = [row(1); row(2); row(3)];

== matlab function Do_Model/Wrench Calculation/Angular Drag/Create Rotation Matrix ==
  data: inverse output; angularPosition input; rotation output
function [inverse, rotation] = fcn(angularPosition)

rotation = eul2rotm([deg2rad(angularPosition(1)), deg2rad(angularPosition(2)), deg2rad(angularPosition(3))]);
inverse = transpose(rotation);

== matlab function Do_Model/Wrench Calculation/Angular Drag/Seperate to Components ==
  data: roll output; pitch output; yaw output; robotFrameVelocity input
function [roll, pitch, yaw] = fcn(robotFrameVelocity)

roll = robotFrameVelocity(1, 1);
pitch = robotFrameVelocity(2, 1);
yaw = robotFrameVelocity(3, 1);

== matlab function Do_Model/Wrench Calculation/Angular Drag/Seperate to World Compents ==
  data: roll output; robotFrameVelocity input; pitch output; yaw output
function [roll, pitch, yaw] = fcn(robotFrameVelocity)

roll = robotFrameVelocity(1, 1);
pitch = robotFrameVelocity(2, 1);
yaw = robotFrameVelocity(3, 1);

== matlab function Do_Model/Wrench Calculation/Thruster Forces and Moments/HSF Thruster/Euler to Unit ==
  data: euler input; direction output
function direction = fcn(euler)

directionCol = eul2rotm(euler, "XYZ") * [1; 0; 0];
direction = [directionCol(1,1), directionCol(2,1), directionCol(3,1)];
